simulink model "Senorless"  (R2023a)
settings: Solver=FixedStepDiscrete  StartTime=0.0  StopTime=5  FixedStep=1/FOC_FRQ  RelTol=1e-3
values from neighbouring files (symbols this model uses):
  ADC_REF = 3.6    [Senorless.sldd]
  ADC_SAMPLE_MAX = 32767.0    [Senorless.sldd]
  AMP_GAIN = 16.0    [Senorless.sldd]
  CURR_INPUT = 3276.0    [Senorless.sldd]
  CURR_KI = 380.0    [Senorless.sldd]
  CURR_KP = 0.04    [Senorless.sldd]
  CURR_LIMIT = 0.95    [Senorless.sldd]
  CURR_OVER = 6.0    [Senorless.sldd]
  CURR_POINT_GAIN = 7.0    [Senorless.sldd]
  CURR_STEP = 32760.0    [Senorless.sldd]
  CURR_UNDER = 0.03    [Senorless.sldd]
  CURR_WIDTH = 6552.0    [Senorless.sldd]
  FOC_FRQ = 25000.0    [Senorless.sldd]
  GAMMA = 32767.0    [Senorless.sldd]
  IMAX = 10.0    [Senorless.sldd]
  LPF_FRQ = 2000.0    [Senorless.sldd]
  MOTOR_DAMPER = 2.06E-7    [Senorless.sldd]
  MOTOR_FLUX = 0.00212352    [Senorless.sldd]
  MOTOR_INERTIA = 4.0E-7    [Senorless.sldd]
  MOTOR_LS = 0.000536    [Senorless.sldd]
  MOTOR_PN = 7.0    [Senorless.sldd]
  MOTOR_RS = 4.0    [Senorless.sldd]
  OPEN_IQ = 0.28    [Senorless.sldd]
  OPEN_IQ_MIN = 0.05    [Senorless.sldd]
  OPEN_IQ_SLOW = 0.1    [Senorless.sldd]
  OPEN_SPD = 1000.0    [Senorless.sldd]
  OPEN_SPD_SLOW = 180.0    [Senorless.sldd]
  OPEN_TIME = 0.5    [Senorless.sldd]
  OPEN_TIME_NFO = 0.5    [Senorless.sldd]
  PLL_LIMIT = 0.9    [Senorless.sldd]
  PLL_WIDTH = 800.0    [Senorless.sldd]
  PWM_FRQ = 96000000.0    [Senorless.sldd]
  RS_HUNT = 0.02    [Senorless.sldd]
  SMOK_FRQ = 600.0    [Senorless.sldd]
  SPD_LIMIT = 0.9    [Senorless.sldd]
  SPD_LPF_LEVEL = 0.0    [Senorless.sldd]
  SPD_MAX = 12000.0    [Senorless.sldd]
  SPD_MIN = 4000.0    [Senorless.sldd]
  SPD_REDUCE = 380.0    [Senorless.sldd]
  SPD_STEP = 6.0    [Senorless.sldd]
  SPD_WIDTH = 20.0    [Senorless.sldd]
  THETA_ERR_LIMIT = 8192.0    [Senorless.sldd]
  TS_POINT_GAIN = 10.0    [Senorless.sldd]
  UDC = 48.0    [Senorless.sldd]
  UDC_GAIN = 21.0    [Senorless.sldd]
  UDC_POINT_GAIN = 10.0    [Senorless.sldd]
undefined symbols (not defined in the file or in its folder): curr_q_ki, curr_q_kp, DiscIntNeverNeededParam, magnitude, PLL_LPF_LEVEL, Udc
libraries: simulink x20, slpidlib x5, mcbcontrolslib x2, mcbplantlib x1, autolibpmsmexterior x1, spspowerguiLib x1
(part 6 of 8)

== system Senorless/FOC_PointModel/恒速降力矩强拖/FreqGenerator_point2 ==
  Freq : Inport
  Xo : Inport  Port=2
  Reset : Inport  Port=3
  Data Type Conversion : DataTypeConversion  OutDataTypeStr=int16  SaturateOnIntegerOverflow=off
  Data Type Conversion1 : DataTypeConversion  OutDataTypeStr=int32  SaturateOnIntegerOverflow=off
  Data Type Conversion2 : DataTypeConversion  OutDataTypeStr=int32  SaturateOnIntegerOverflow=off
  Discrete-Time Integrator : DiscreteIntegrator  ExternalReset=falling  InitialConditionSource=external  SampleTime=-1  OutDataTypeStr=int32  RndMeth=Zero  ICPrevOutput=DiscIntNeverNeededParam  ICPrevScaledInput=DiscIntNeverNeededParam
  Gain6 : Gain  Gain=65535  OutDataTypeStr=int32
  MATLAB Function1 : MATLAB Function  Commented=on  TreatAsAtomicUnit=on
  Scope : Scope
  Shift Arithmetic : ArithShift  BitShiftNumber=-8
  Shift Arithmetic1 : ArithShift  BitShiftNumber=8
  Shift Arithmetic2 : ArithShift  BitShiftNumber=-8
  Theta : Outport
  wires:
  Shift Arithmetic/1 -> Discrete-Time Integrator/1
  Freq/1 -> Data Type Conversion1/1
  Gain6/1 -> Shift Arithmetic/1
  Data Type Conversion1/1 -> Gain6/1
  Shift Arithmetic1/1 -> Data Type Conversion/1
  Data Type Conversion/1 -> Theta/1
  Data Type Conversion2/1 -> Shift Arithmetic2/1
  Discrete-Time Integrator/1 -> Scope/1, Shift Arithmetic1/1
  Xo/1 -> Data Type Conversion2/1
  Shift Arithmetic2/1 -> Discrete-Time Integrator/3
  Reset/1 -> Discrete-Time Integrator/2

== system Senorless/FOC_PointModel/恒速降力矩强拖/积分器 ==
  input : Inport
  Xo : Inport  Port=2
  Constant : Constant  OutDataTypeStr=int16
  Data Store Read1 : DataStoreRead  DataStoreName=Ts_Point  IndexOptions=Index vector (dialog)  Indices=1  OutputSizes=1
  Delay : Delay  DelayLength=1  InitialConditionSource=Input port
      settings: InputPortMap=u0,p4
  Product1 : Product  OutDataTypeStr=int32  RndMeth=Zero
  Product2 : Product  OutDataTypeStr=int32  RndMeth=Zero
  Shift Arithmetic : ArithShift  BitShiftNumberSource=Input port  BitShiftNumber=8  BitShiftDirection=Right
      settings: InputPortMap=u0,p1
  Sum : Sum  Inputs=|++  OutDataTypeStr=int32  RndMeth=Zero
  周期定点化适当放大2^n : Constant  Value=TS_POINT_GAIN
  这个是缩小周期增益的 : ArithShift  BitShiftNumber=15  DiagnosticForOORShift=Error
  output : Outport
  wires:
  Sum/1 -> Delay/1, output/1
  Product2/1 -> 这个是缩小周期增益的/1
  input/1 -> Shift Arithmetic/1
  Data Store Read1/1 -> Product2/1
  Shift Arithmetic/1 -> Product2/2
  周期定点化适当放大2^n/1 -> Shift Arithmetic/2
  Xo/1 -> Delay/2
  这个是缩小周期增益的/1 -> Product1/1
  Constant/1 -> Product1/2
  Product1/1 -> Sum/1
  Delay/1 -> Sum/2

== system Senorless/FOC_PointModel/慢速开环/FreqGenerator_point2 ==
  Freq : Inport
  Xo : Inport  Port=2
  Reset : Inport  Port=3
  Data Type Conversion : DataTypeConversion  OutDataTypeStr=int16  SaturateOnIntegerOverflow=off
  Data Type Conversion1 : DataTypeConversion  OutDataTypeStr=int32  SaturateOnIntegerOverflow=off
  Data Type Conversion2 : DataTypeConversion  OutDataTypeStr=int32  SaturateOnIntegerOverflow=off
  Discrete-Time Integrator : DiscreteIntegrator  ExternalReset=falling  InitialConditionSource=external  SampleTime=-1  OutDataTypeStr=int32  RndMeth=Zero  ICPrevOutput=DiscIntNeverNeededParam  ICPrevScaledInput=DiscIntNeverNeededParam
  Gain6 : Gain  Gain=65535  OutDataTypeStr=int32
  MATLAB Function1 : MATLAB Function  Commented=on  TreatAsAtomicUnit=on
  Scope : Scope
  Shift Arithmetic : ArithShift  BitShiftNumber=-8
  Shift Arithmetic1 : ArithShift  BitShiftNumber=8
  Shift Arithmetic2 : ArithShift  BitShiftNumber=-8
  Theta : Outport
  wires:
  Reset/1 -> Discrete-Time Integrator/2
  Shift Arithmetic2/1 -> Discrete-Time Integrator/3
  Xo/1 -> Data Type Conversion2/1
  Discrete-Time Integrator/1 -> Shift Arithmetic1/1, Scope/1
  Data Type Conversion2/1 -> Shift Arithmetic2/1
  Data Type Conversion/1 -> Theta/1
  Shift Arithmetic1/1 -> Data Type Conversion/1
  Data Type Conversion1/1 -> Gain6/1
  Gain6/1 -> Shift Arithmetic/1
  Freq/1 -> Data Type Conversion1/1
  Shift Arithmetic/1 -> Discrete-Time Integrator/1

== system Senorless/FOC_PointModel/慢速开环/积分器 ==
  input : Inport
  Constant : Constant  OutDataTypeStr=int16
  Data Store Read1 : DataStoreRead  DataStoreName=Ts_Point  IndexOptions=Index vector (dialog)  Indices=1  OutputSizes=1
  Product1 : Product  OutDataTypeStr=int32  RndMeth=Zero
  Product2 : Product  OutDataTypeStr=int32  RndMeth=Zero
  Shift Arithmetic : ArithShift  BitShiftNumberSource=Input port  BitShiftNumber=8  BitShiftDirection=Right
      settings: InputPortMap=u0,p1
  Sum : Sum  Inputs=|++  OutDataTypeStr=int32  RndMeth=Zero
  Unit Delay : UnitDelay  SampleTime=-1  HasFrameUpgradeWarning=on
  周期定点化适当放大2^n : Constant  Value=TS_POINT_GAIN
  这个是缩小周期增益的 : ArithShift  BitShiftNumber=15  DiagnosticForOORShift=Error
  output : Outport
  wires:
  周期定点化适当放大2^n/1 -> Shift Arithmetic/2
  Shift Arithmetic/1 -> Product2/2
  Data Store Read1/1 -> Product2/1
  input/1 -> Shift Arithmetic/1
  这个是缩小周期增益的/1 -> Product1/2
  Product2/1 -> 这个是缩小周期增益的/1
  Product1/1 -> Sum/1
  Sum/1 -> Unit Delay/1, output/1
  Unit Delay/1 -> Sum/2
  Constant/1 -> Product1/1

== system Senorless/FOC_PointModel/观测器闭环//速度环/PI Controller ==
  input : Inport
  Kp : Inport  Port=2
  Ki : Inport  Port=3
  Data Store Read3 : DataStoreRead  DataStoreName=Speed_Limit  IndexOptions=Index vector (dialog)  Indices=1  OutputSizes=1
  Gain : Gain  Gain=-1  OutDataTypeStr=int32  RndMeth=Zero
  Product2 : Product  OutDataTypeStr=int32  RndMeth=Zero
  Saturation Dynamic2 : simulink/Discontinuities/Saturation Dynamic  OutMin=[]  OutMax=[]  OutDataTypeStr=Inherit: Same as second input  OutDataType=fixdt(1, 16)  OutScaling=2^-10  RndMeth=Zero  DoSatur=off
  Scope : Scope  NumInputPorts=2
  Scope1 : Scope  NumInputPorts=2
  Sum : Sum  OutDataTypeStr=int32  RndMeth=Zero
  input1 : InportShadow
  积分器 : Subsystem  Commented=on
      settings: MinAlgLoopOccurrences=on
  output : Outport
  wires:
  input/1 -> Scope1/1, Product2/1
  input1/1 -> 积分器/2(input)
  Sum/1 -> Saturation Dynamic2/2
  Saturation Dynamic2/1 -> output/1
  Data Store Read3/1 -> [limit]
  [limit] -> Gain/1
  Product2/1 -> Scope1/2, Sum/1, Scope/1
  积分器/1(output) -> Scope/2
  Kp/1 -> Product2/2
  Ki/1 -> 积分器/1(Ki)
  Gain/1 -> Saturation Dynamic2/3
  [limit] -> Saturation Dynamic2/1

== system Senorless/FOC_PointModel/观测器闭环//速度环/积分器//上升沿初始化 ==
  Ki : Inport
  input : Inport  Port=2
  Reset : Inport  Port=3
  Xo : Inport  Port=4
  Data Store Memory : DataStoreMemory  DataStoreName=tmp  WriteAfterWriteMsg=warning  ShowAdditionalParam=off  OutDataTypeStr=int32
  Data Store Read : DataStoreRead  DataStoreName=tmp  IndexOptions=Index vector (dialog)  Indices=1  OutputSizes=1
  Data Store Read1 : DataStoreRead  DataStoreName=Ts_Point  IndexOptions=Index vector (dialog)  Indices=1  OutputSizes=1
  Data Store Write : DataStoreWrite  DataStoreName=tmp  IndexOptions=Index vector (dialog)  Indices=1  OutputSizes=1
  Data Type Conversion2 : DataTypeConversion  OutDataTypeStr=int32  SaturateOnIntegerOverflow=off
  Data Type Conversion3 : DataTypeConversion  Commented=on  OutDataTypeStr=int16  SaturateOnIntegerOverflow=off
  Divide : Product  Commented=on  Inputs=*/  OutDataTypeStr=int32  RndMeth=Zero
  MATLAB Function : MATLAB Function  TreatAsAtomicUnit=on
  Product1 : Product  OutDataTypeStr=int32  RndMeth=Zero
  Product2 : Product  OutDataTypeStr=int32  RndMeth=Zero
  Reset_Block : Subsystem
  Scope : Scope
  Sum : Sum  Inputs=|++  OutDataTypeStr=int32  RndMeth=Zero
  Sum1 : Sum  Inputs=|+-  OutDataTypeStr=int32  RndMeth=Zero
  Ts适当放大的缩小系数， 详见初始化模块 : ArithShift  Commented=on  BitShiftNumber=TS_POINT_GAIN  DiagnosticForOORShift=Error
  Unit Delay : UnitDelay  SampleTime=-1  HasFrameUpgradeWarning=on
  周期定点化适当放大2^n : Constant  Value=TS_POINT_GAIN
  积分器运行频率 : Constant  Commented=on  Value=FOC_FRQ
  这个是缩小周期增益的 : ArithShift  BitShiftNumber=15  DiagnosticForOORShift=Error
  output : Outport
  wires:
  周期定点化适当放大2^n/1 -> MATLAB Function/2(n)
  Sum1/1 -> Reset_Block/1(Xo)
  MATLAB Function/1(out) -> Product2/2
  Data Store Read1/1 -> Product2/1
  input/1 -> MATLAB Function/1(in)
  这个是缩小周期增益的/1 -> Product1/2
  Product2/1 -> 这个是缩小周期增益的/1
  Data Type Conversion3/1 -> Divide/2
  Ki/1 -> Product1/1
  Xo/1 -> Data Type Conversion2/1
  积分器运行频率/1 -> Data Type Conversion3/1
  Product1/1 -> Sum/1, Sum1/2
  Data Type Conversion2/1 -> Sum1/1
  Unit Delay/1 -> Data Store Write/1
  Sum/1 -> output/1, Scope/1, Unit Delay/1
  Data Store Read/1 -> Sum/2
  Reset/1 -> Reset_Block/Trigger

== system Senorless/FOC_PointModel/Err/闭环错误判断/SUM ==
  in : Inport
  Action Port : ActionPort  InitializeStates=reset  ActionPortLabel=if(u1 > 0)
  Sum : Sum  Inputs=|++  OutDataTypeStr=int32  RndMeth=Zero
  Unit Delay2 : UnitDelay  SampleTime=-1  HasFrameUpgradeWarning=on
  out : Outport
  wires:
  Sum/1 -> Unit Delay2/1
  in/1 -> Sum/1
  Unit Delay2/1 -> out/1, Sum/2

== system Senorless/FOC_PointModel/Err/闭环错误判断/ZERO ==
  Action Port : ActionPort  InitializeStates=reset  ActionPortLabel=else
  Constant : Constant  Value=0  OutDataTypeStr=int32
  out : Outport
  wires:
  Constant/1 -> out/1

== system Senorless/FOC_PointModel/Observers/PLL/LPF ==
  note: a =(ω c​ T s​ )/(1+ω c​ T s​ )
  note: y(n)=ax(n)+(1−a)y(n−1)
  input : Inport
  Constant1 : Constant  Value=SPD_LPF_LEVEL  OutDataTypeStr=int16
  Constant5 : Constant  OutDataTypeStr=int16
  Product10 : Product  OutDataTypeStr=int32
  Product11 : Product  OutDataTypeStr=int32  RndMeth=Zero
  Saturation : Saturate  UpperLimit=15  LowerLimit=0  RndMeth=Zero
  Shift Arithmetic1 : ArithShift  BitShiftNumber=-4
  Shift Arithmetic9 : ArithShift  BitShiftNumber=4
  Sum10 : Sum  Inputs=-+
  Sum11 : Sum  OutDataTypeStr=int32  RndMeth=Zero
  Unit Delay9 : UnitDelay  SampleTime=-1  HasFrameUpgradeWarning=on
  output : Outport
  wires:
  Constant1/1 -> Saturation/1
  Constant5/1 -> Shift Arithmetic1/1
  Sum11/1 -> Shift Arithmetic9/1
  Shift Arithmetic9/1 -> output/1, Unit Delay9/1
  Shift Arithmetic1/1 -> Sum10/2
  Sum10/1 -> Product10/1
  Product11/1 -> Sum11/1
  Product10/1 -> Sum11/2
  Unit Delay9/1 -> Product11/1
  input/1 -> Product10/2
  Saturation/1 -> Sum10/1, Product11/2

== system Senorless/FOC_PointModel/Observers/PLL/PI Controller ==
  input : Inport
  Kp : Inport  Port=2
  Ki : Inport  Port=3
  Data Store Read3 : DataStoreRead  DataStoreName=PLL_Limit  IndexOptions=Index vector (dialog)  Indices=1  OutputSizes=1
  Gain : Gain  Gain=-1  OutDataTypeStr=int32  RndMeth=Zero
  Product2 : Product  OutDataTypeStr=int32  RndMeth=Zero
  Saturation Dynamic2 : simulink/Discontinuities/Saturation Dynamic  OutMin=[]  OutMax=[]  OutDataTypeStr=Inherit: Same as second input  OutDataType=fixdt(1, 16)  OutScaling=2^-10  RndMeth=Zero  DoSatur=off
  Scope : Scope  NumInputPorts=2
  Sum : Sum  OutDataTypeStr=int32  RndMeth=Zero
  input1 : InportShadow
  积分器 : Subsystem
      settings: MinAlgLoopOccurrences=on
  output : Outport
  wires:
  input/1 -> Product2/1
  Kp/1 -> Product2/2
  Ki/1 -> 积分器/1(Ki)
  input1/1 -> 积分器/2(input)
  Product2/1 -> Sum/1, Scope/1
  积分器/1(output) -> Scope/2, Sum/2
  Saturation Dynamic2/1 -> output/1
  Data Store Read3/1 -> [Limit]
  [Limit] -> Gain/1
  Gain/1 -> Saturation Dynamic2/3
  Sum/1 -> Saturation Dynamic2/2
  [Limit] -> Saturation Dynamic2/1

== system Senorless/FOC_PointModel/Observers/PLL/PLL_LPF1 ==
  note: y(n)=ax(n)+(1−a)y(n−1)
  note: a =(ω c​ T s​ )/(1+ω c​ T s​ )
  input : Inport
  Constant1 : Constant  Value=PLL_LPF_LEVEL  OutDataTypeStr=int16
  Constant5 : Constant  OutDataTypeStr=int16
  Product10 : Product  OutDataTypeStr=int32
  Product11 : Product  OutDataTypeStr=int32  RndMeth=Zero
  Shift Arithmetic1 : ArithShift  BitShiftNumber=-4
  Shift Arithmetic9 : ArithShift  BitShiftNumber=4
  Sum10 : Sum  Inputs=-+
  Sum11 : Sum  OutDataTypeStr=int32  RndMeth=Zero
  Unit Delay9 : UnitDelay  SampleTime=-1  HasFrameUpgradeWarning=on
  output : Outport
  wires:
  input/1 -> Product10/2
  Unit Delay9/1 -> Product11/1
  Product10/1 -> Sum11/2
  Product11/1 -> Sum11/1
  Sum10/1 -> Product10/1
  Shift Arithmetic1/1 -> Sum10/2
  Shift Arithmetic9/1 -> Unit Delay9/1, output/1
  Sum11/1 -> Shift Arithmetic9/1
  Constant5/1 -> Shift Arithmetic1/1
  Constant1/1 -> Product11/2, Sum10/1

== system Senorless/FOC_PointModel/Observers/PLL/sincos_512 ==
  theta : Inport
  Constant3 : Constant  Value=16384  OutDataTypeStr=uint16
  Shift Arithmetic : ArithShift  BitShiftNumber=7
  Shift Arithmetic1 : ArithShift  BitShiftNumber=7
  Sin : Lookup_n-D  NumberOfTableDimensions=1  BreakpointsSpecification=Even spacing  BreakpointsForDimension1=uint16(linspace(0,511,512))  BreakpointsForDimension1DataTypeStr=uint16  IndexSearchMethod=Linear search  BeginIndexSearchUsingPreviousIndexResult=on  UseOneInputPortForAllInputData=on  Table=int16(32767*sin(linspace(0,2*pi,512)))  TableDataTypeStr=int16  IntermediateResultsDataTypeStr=int32  InterpMethod=Flat  ExtrapMethod=Clip  RemoveProtectionInput=on  ApplyFullPrecisionForLinearInterpolation=on  InternalRulePriority=Speed  OutDataTypeStr=int16  RndMeth=Zero  FractionDataTypeStr=fixdt(1,16,0)  InputSameDT=off
  Sin1 : Lookup_n-D  NumberOfTableDimensions=1  BreakpointsSpecification=Even spacing  BreakpointsForDimension1=uint16(linspace(0,511,512))  BreakpointsForDimension1DataTypeStr=uint16  IndexSearchMethod=Linear search  BeginIndexSearchUsingPreviousIndexResult=on  UseOneInputPortForAllInputData=on  Table=int16(32767*sin(linspace(0,2*pi,512)))  TableDataTypeStr=int16  IntermediateResultsDataTypeStr=int32  InterpMethod=Flat  ExtrapMethod=Clip  RemoveProtectionInput=on  ApplyFullPrecisionForLinearInterpolation=on  InternalRulePriority=Speed  OutDataTypeStr=int16  RndMeth=Zero  FractionDataTypeStr=fixdt(1,16,0)  InputSameDT=off
  Sum2 : Sum  Inputs=|++
  theta1 : InportShadow
  cos : Outport
  sin : Outport  Port=2
  wires:
  Sin1/1 -> cos/1
  Sin/1 -> sin/1
  Shift Arithmetic/1 -> Sin1/1
  Sum2/1 -> Shift Arithmetic/1
  Constant3/1 -> Sum2/2
  Shift Arithmetic1/1 -> Sin/1
  theta1/1 -> Sum2/1
  theta/1 -> Shift Arithmetic1/1

== system Senorless/FOC_PointModel/Observers/PLL/积分器 ==
  input : Inport
  Constant : Constant  OutDataTypeStr=int16
  Data Store Read1 : DataStoreRead  DataStoreName=Ts_Point  IndexOptions=Index vector (dialog)  Indices=1  OutputSizes=1
  Data Type Conversion3 : DataTypeConversion  Commented=on  OutDataTypeStr=int16  SaturateOnIntegerOverflow=off
  Divide : Product  Commented=on  Inputs=*/  OutDataTypeStr=int32  RndMeth=Zero
  Product1 : Product  OutDataTypeStr=int32  RndMeth=Zero
  Product2 : Product  OutDataTypeStr=int32  RndMeth=Zero
  Shift Arithmetic : ArithShift  BitShiftNumberSource=Input port  BitShiftNumber=8  BitShiftDirection=Right
      settings: InputPortMap=u0,p1
  Sum : Sum  Inputs=|++  OutDataTypeStr=int32  RndMeth=Zero
  Ts适当放大的缩小系数， 详见初始化模块 : ArithShift  Commented=on  BitShiftNumber=TS_POINT_GAIN  DiagnosticForOORShift=Error
  Unit Delay : UnitDelay  SampleTime=-1  HasFrameUpgradeWarning=on
  周期定点化适当放大2^n : Constant  Value=TS_POINT_GAIN
  积分器运行频率 : Constant  Commented=on  Value=FOC_FRQ
  这个是缩小周期增益的 : ArithShift  BitShiftNumber=15  DiagnosticForOORShift=Error
  output : Outport
  wires:
  积分器运行频率/1 -> Data Type Conversion3/1
  Data Type Conversion3/1 -> Divide/2
  周期定点化适当放大2^n/1 -> Shift Arithmetic/2
  Sum/1 -> output/1, Unit Delay/1
  Unit Delay/1 -> Sum/2
  input/1 -> Shift Arithmetic/1
  Shift Arithmetic/1 -> Product2/2
  Data Store Read1/1 -> Product2/1
  Product2/1 -> 这个是缩小周期增益的/1
  这个是缩小周期增益的/1 -> Product1/2
  Constant/1 -> Product1/1
  Product1/1 -> Sum/1

== system Senorless/FOC_PointModel/Observers/PLL2/LPF ==
  note: y(n)=ax(n)+(1−a)y(n−1)
  note: a =(ω c​ T s​ )/(1+ω c​ T s​ )
  input : Inport
  Constant1 : Constant  Value=8  OutDataTypeStr=int16
  Constant5 : Constant  OutDataTypeStr=int16
  Product10 : Product  OutDataTypeStr=int32
  Product11 : Product  OutDataTypeStr=int32  RndMeth=Zero
  Saturation : Saturate  UpperLimit=15  LowerLimit=0  RndMeth=Zero
  Shift Arithmetic1 : ArithShift  BitShiftNumber=-4
  Shift Arithmetic9 : ArithShift  BitShiftNumber=4
  Sum10 : Sum  Inputs=-+
  Sum11 : Sum  OutDataTypeStr=int32  RndMeth=Zero
  Unit Delay9 : UnitDelay  SampleTime=-1  HasFrameUpgradeWarning=on
  output : Outport
  wires:
  Saturation/1 -> Product11/2, Sum10/1
  input/1 -> Product10/2
  Unit Delay9/1 -> Product11/1
  Product10/1 -> Sum11/2
  Product11/1 -> Sum11/1
  Sum10/1 -> Product10/1
  Shift Arithmetic1/1 -> Sum10/2
  Shift Arithmetic9/1 -> Unit Delay9/1, output/1
  Sum11/1 -> Shift Arithmetic9/1
  Constant5/1 -> Shift Arithmetic1/1
  Constant1/1 -> Saturation/1

== system Senorless/FOC_PointModel/Observers/PLL2/PI Controller ==
  input : Inport
  Kp : Inport  Port=2
  Ki : Inport  Port=3
  Data Store Read3 : DataStoreRead  DataStoreName=PLL_Limit  IndexOptions=Index vector (dialog)  Indices=1  OutputSizes=1
  Gain : Gain  Gain=-1  OutDataTypeStr=int32  RndMeth=Zero
  Product2 : Product  OutDataTypeStr=int32  RndMeth=Zero
  Saturation Dynamic2 : simulink/Discontinuities/Saturation Dynamic  OutMin=[]  OutMax=[]  OutDataTypeStr=Inherit: Same as second input  OutDataType=fixdt(1, 16)  OutScaling=2^-10  RndMeth=Zero  DoSatur=off
  Scope : Scope  NumInputPorts=2
  Sum : Sum  OutDataTypeStr=int32  RndMeth=Zero
  input1 : InportShadow
  积分器 : Subsystem
      settings: MinAlgLoopOccurrences=on
  output : Outport
  wires:
  [Limit] -> Saturation Dynamic2/1
  Sum/1 -> Saturation Dynamic2/2
  Gain/1 -> Saturation Dynamic2/3
  [Limit] -> Gain/1
  Data Store Read3/1 -> [Limit]
  Saturation Dynamic2/1 -> output/1
  积分器/1(output) -> Sum/2, Scope/2
  Product2/1 -> Scope/1, Sum/1
  input1/1 -> 积分器/2(input)
  Ki/1 -> 积分器/1(Ki)
  Kp/1 -> Product2/2
  input/1 -> Product2/1

== system Senorless/FOC_PointModel/Observers/PLL2/PLL_LPF1 ==
  note: a =(ω c​ T s​ )/(1+ω c​ T s​ )
  note: y(n)=ax(n)+(1−a)y(n−1)
  input : Inport
  Constant1 : Constant  Value=PLL_LPF_LEVEL  OutDataTypeStr=int16
  Constant5 : Constant  OutDataTypeStr=int16
  Product10 : Product  OutDataTypeStr=int32
  Product11 : Product  OutDataTypeStr=int32  RndMeth=Zero
  Shift Arithmetic1 : ArithShift  BitShiftNumber=-4
  Shift Arithmetic9 : ArithShift  BitShiftNumber=4
  Sum10 : Sum  Inputs=-+
  Sum11 : Sum  OutDataTypeStr=int32  RndMeth=Zero
  Unit Delay9 : UnitDelay  SampleTime=-1  HasFrameUpgradeWarning=on
  output : Outport
  wires:
  Constant1/1 -> Sum10/1, Product11/2
  Constant5/1 -> Shift Arithmetic1/1
  Sum11/1 -> Shift Arithmetic9/1
  Shift Arithmetic9/1 -> output/1, Unit Delay9/1
  Shift Arithmetic1/1 -> Sum10/2
  Sum10/1 -> Product10/1
  Product11/1 -> Sum11/1
  Product10/1 -> Sum11/2
  Unit Delay9/1 -> Product11/1
  input/1 -> Product10/2

== system Senorless/FOC_PointModel/Observers/PLL2/sincos_512 ==
  theta : Inport
  Constant3 : Constant  Value=16384  OutDataTypeStr=uint16
  Shift Arithmetic : ArithShift  BitShiftNumber=7
  Shift Arithmetic1 : ArithShift  BitShiftNumber=7
  Sin : Lookup_n-D  NumberOfTableDimensions=1  BreakpointsSpecification=Even spacing  BreakpointsForDimension1=uint16(linspace(0,511,512))  BreakpointsForDimension1DataTypeStr=uint16  IndexSearchMethod=Linear search  BeginIndexSearchUsingPreviousIndexResult=on  UseOneInputPortForAllInputData=on  Table=int16(32767*sin(linspace(0,2*pi,512)))  TableDataTypeStr=int16  IntermediateResultsDataTypeStr=int32  InterpMethod=Flat  ExtrapMethod=Clip  RemoveProtectionInput=on  ApplyFullPrecisionForLinearInterpolation=on  InternalRulePriority=Speed  OutDataTypeStr=int16  RndMeth=Zero  FractionDataTypeStr=fixdt(1,16,0)  InputSameDT=off
  Sin1 : Lookup_n-D  NumberOfTableDimensions=1  BreakpointsSpecification=Even spacing  BreakpointsForDimension1=uint16(linspace(0,511,512))  BreakpointsForDimension1DataTypeStr=uint16  IndexSearchMethod=Linear search  BeginIndexSearchUsingPreviousIndexResult=on  UseOneInputPortForAllInputData=on  Table=int16(32767*sin(linspace(0,2*pi,512)))  TableDataTypeStr=int16  IntermediateResultsDataTypeStr=int32  InterpMethod=Flat  ExtrapMethod=Clip  RemoveProtectionInput=on  ApplyFullPrecisionForLinearInterpolation=on  InternalRulePriority=Speed  OutDataTypeStr=int16  RndMeth=Zero  FractionDataTypeStr=fixdt(1,16,0)  InputSameDT=off
  Sum2 : Sum  Inputs=|++
  theta1 : InportShadow
  cos : Outport
  sin : Outport  Port=2
  wires:
  theta/1 -> Shift Arithmetic1/1
  theta1/1 -> Sum2/1
  Shift Arithmetic1/1 -> Sin/1
  Constant3/1 -> Sum2/2
  Sum2/1 -> Shift Arithmetic/1
  Shift Arithmetic/1 -> Sin1/1
  Sin/1 -> sin/1
  Sin1/1 -> cos/1

== system Senorless/FOC_PointModel/Observers/PLL2/积分器 ==
  input : Inport
  Constant : Constant  OutDataTypeStr=int16
  Data Store Read1 : DataStoreRead  DataStoreName=Ts_Point  IndexOptions=Index vector (dialog)  Indices=1  OutputSizes=1
  Data Type Conversion3 : DataTypeConversion  Commented=on  OutDataTypeStr=int16  SaturateOnIntegerOverflow=off
  Divide : Product  Commented=on  Inputs=*/  OutDataTypeStr=int32  RndMeth=Zero
  Product1 : Product  OutDataTypeStr=int32  RndMeth=Zero
  Product2 : Product  OutDataTypeStr=int32  RndMeth=Zero
  Shift Arithmetic : ArithShift  BitShiftNumberSource=Input port  BitShiftNumber=8  BitShiftDirection=Right
      settings: InputPortMap=u0,p1
  Sum : Sum  Inputs=|++  OutDataTypeStr=int32  RndMeth=Zero
  Ts适当放大的缩小系数， 详见初始化模块 : ArithShift  Commented=on  BitShiftNumber=TS_POINT_GAIN  DiagnosticForOORShift=Error
  Unit Delay : UnitDelay  SampleTime=-1  HasFrameUpgradeWarning=on
  周期定点化适当放大2^n : Constant  Value=TS_POINT_GAIN
  积分器运行频率 : Constant  Commented=on  Value=FOC_FRQ
  这个是缩小周期增益的 : ArithShift  BitShiftNumber=15  DiagnosticForOORShift=Error
  output : Outport
  wires:
  Product1/1 -> Sum/1
  Constant/1 -> Product1/1
  这个是缩小周期增益的/1 -> Product1/2
  Product2/1 -> 这个是缩小周期增益的/1
  Data Store Read1/1 -> Product2/1
  Shift Arithmetic/1 -> Product2/2
  input/1 -> Shift Arithmetic/1
  Unit Delay/1 -> Sum/2
  Sum/1 -> Unit Delay/1, output/1
  周期定点化适当放大2^n/1 -> Shift Arithmetic/2
  Data Type Conversion3/1 -> Divide/2
  积分器运行频率/1 -> Data Type Conversion3/1

== system Senorless/FOC_PointModel/Observers/SMO/SMO_LPF1 ==
  note: y(n)=ax(n)+(1−a)y(n−1)
  note: a =(ω c​ T s​ )/(1+ω c​ T s​ )
  input : Inport
  Constant5 : Constant  Value=32767  OutDataTypeStr=int16
  Data Store Read1 : DataStoreRead  DataStoreName=LPF_FRQ_Point  IndexOptions=Index vector (dialog)  Indices=1  OutputSizes=1
  Data Store Read7 : DataStoreRead  DataStoreName=LPF_FRQ_Point  IndexOptions=Index vector (dialog)  Indices=1  OutputSizes=1
  Product1 : Product  OutDataTypeStr=int32  RndMeth=Zero
  Product10 : Product  OutDataTypeStr=int32
  Product11 : Product  OutDataTypeStr=int32  RndMeth=Zero
  Shift Arithmetic2 : ArithShift  BitShiftNumber=15
  Shift Arithmetic3 : ArithShift  BitShiftNumber=15
  Shift Arithmetic4 : ArithShift  BitShiftNumber=15
  Sum1 : Sum  Inputs=-+  OutDataTypeStr=int32  RndMeth=Zero
  Sum10 : Sum  Inputs=-+  OutDataTypeStr=int16  RndMeth=Zero
  Sum11 : Sum  OutDataTypeStr=int32  RndMeth=Zero
  Sum2 : Sum  OutDataTypeStr=int32  RndMeth=Zero
  Unit Delay1 : UnitDelay  SampleTime=-1  HasFrameUpgradeWarning=on
  Unit Delay9 : UnitDelay  SampleTime=-1  HasFrameUpgradeWarning=on
  input1 : InportShadow
  output : Outport
  wires:
  Product10/1 -> Shift Arithmetic3/1
  Product11/1 -> Shift Arithmetic2/1
  Unit Delay9/1 -> Product10/2
  Sum10/1 -> Product10/1
  input/1 -> Product11/1
  Data Store Read7/1 -> Sum10/1, Product11/2
  Sum11/1 -> Unit Delay9/1
  Shift Arithmetic2/1 -> Sum11/1
  Shift Arithmetic3/1 -> Sum11/2
  input1/1 -> Sum1/2
  Unit Delay1/1 -> Sum2/1, Sum1/1
  Sum2/1 -> output/1, Unit Delay1/1
  Sum1/1 -> Product1/1
  Data Store Read1/1 -> Product1/2
  Product1/1 -> Shift Arithmetic4/1
  Shift Arithmetic4/1 -> Sum2/2
  Constant5/1 -> Sum10/2

== system Senorless/FOC_PointModel/Observers/SMO/SMO_LPF2 ==
  note: a =(ω c​ T s​ )/(1+ω c​ T s​ )
  note: y(n)=ax(n)+(1−a)y(n−1)
  input : Inport
  Constant5 : Constant  Value=32767  OutDataTypeStr=int16
  Data Store Read1 : DataStoreRead  DataStoreName=LPF_FRQ_Point  IndexOptions=Index vector (dialog)  Indices=1  OutputSizes=1
  Data Store Read7 : DataStoreRead  DataStoreName=LPF_FRQ_Point  IndexOptions=Index vector (dialog)  Indices=1  OutputSizes=1
  Product1 : Product  OutDataTypeStr=int32  RndMeth=Zero
  Product10 : Product  OutDataTypeStr=int32
  Product11 : Product  OutDataTypeStr=int32  RndMeth=Zero
  Shift Arithmetic2 : ArithShift  BitShiftNumber=15
  Shift Arithmetic3 : ArithShift  BitShiftNumber=15
  Shift Arithmetic4 : ArithShift  BitShiftNumber=15
  Sum1 : Sum  Inputs=-+  OutDataTypeStr=int32  RndMeth=Zero
  Sum10 : Sum  Inputs=-+  OutDataTypeStr=int16  RndMeth=Zero
  Sum11 : Sum  OutDataTypeStr=int32  RndMeth=Zero
  Sum2 : Sum  OutDataTypeStr=int32  RndMeth=Zero
  Unit Delay1 : UnitDelay  SampleTime=-1  HasFrameUpgradeWarning=on
  Unit Delay9 : UnitDelay  SampleTime=-1  HasFrameUpgradeWarning=on
  input1 : InportShadow
  output : Outport
  wires:
  Shift Arithmetic4/1 -> Sum2/2
  Product1/1 -> Shift Arithmetic4/1
  Data Store Read1/1 -> Product1/2
  Sum1/1 -> Product1/1
  Sum2/1 -> output/1, Unit Delay1/1
  Unit Delay1/1 -> Sum1/1, Sum2/1
  input1/1 -> Sum1/2
  Shift Arithmetic3/1 -> Sum11/2
  Shift Arithmetic2/1 -> Sum11/1
  Data Store Read7/1 -> Product11/2, Sum10/1
  Constant5/1 -> Sum10/2
  input/1 -> Product11/1
  Sum10/1 -> Product10/1
  Unit Delay9/1 -> Product10/2
  Product11/1 -> Shift Arithmetic2/1
  Product10/1 -> Shift Arithmetic3/1
  Sum11/1 -> Unit Delay9/1

== system Senorless/FOC_PointModel/Observers/SMO/SMO_LPF4 ==
  note: a =(ω c​ T s​ )/(1+ω c​ T s​ )
  note: y(n)=ax(n)+(1−a)y(n−1)
  input : Inport
  Constant5 : Constant  OutDataTypeStr=int16
  Data Store Read7 : DataStoreRead  DataStoreName=LPF_FRQ_Point  IndexOptions=Index vector (dialog)  Indices=1  OutputSizes=1
  Data Type Conversion6 : DataTypeConversion  OutDataTypeStr=int16  SaturateOnIntegerOverflow=off
  Product10 : Product  OutDataTypeStr=int32
  Product11 : Product  OutDataTypeStr=int32  RndMeth=Zero
  Shift Arithmetic1 : ArithShift  BitShiftNumber=-4
  Shift Arithmetic9 : ArithShift  BitShiftNumber=4
  Sum10 : Sum  Inputs=-+
  Sum11 : Sum  OutDataTypeStr=int32  RndMeth=Zero
  Unit Delay9 : UnitDelay  SampleTime=-1  HasFrameUpgradeWarning=on
  output : Outport
  wires:
  Constant5/1 -> Shift Arithmetic1/1
  Sum11/1 -> Shift Arithmetic9/1
  Data Type Conversion6/1 -> output/1, Unit Delay9/1
  Shift Arithmetic9/1 -> Data Type Conversion6/1
  Data Store Read7/1 -> Product11/2, Sum10/1
  Shift Arithmetic1/1 -> Sum10/2
  input/1 -> Product11/1
  Sum10/1 -> Product10/1
  Unit Delay9/1 -> Product10/2
  Product11/1 -> Sum11/1
  Product10/1 -> Sum11/2

== system Senorless/FOC_PointModel/Observers/SMO/SMO_LPF5 ==
  note: y(n)=ax(n)+(1−a)y(n−1)
  note: a =(ω c​ T s​ )/(1+ω c​ T s​ )
  input : Inport
  Constant5 : Constant  OutDataTypeStr=int16
  Data Store Read7 : DataStoreRead  DataStoreName=LPF_FRQ_Point  IndexOptions=Index vector (dialog)  Indices=1  OutputSizes=1
  Data Type Conversion6 : DataTypeConversion  OutDataTypeStr=int16  SaturateOnIntegerOverflow=off
  Product10 : Product  OutDataTypeStr=int32
  Product11 : Product  OutDataTypeStr=int32  RndMeth=Zero
  Shift Arithmetic1 : ArithShift  BitShiftNumber=-4
  Shift Arithmetic9 : ArithShift  BitShiftNumber=4
  Sum10 : Sum  Inputs=-+
  Sum11 : Sum  OutDataTypeStr=int32  RndMeth=Zero
  Unit Delay9 : UnitDelay  SampleTime=-1  HasFrameUpgradeWarning=on
  output : Outport
  wires:
  Product10/1 -> Sum11/2
  Product11/1 -> Sum11/1
  Unit Delay9/1 -> Product10/2
  Sum10/1 -> Product10/1
  input/1 -> Product11/1
  Shift Arithmetic1/1 -> Sum10/2
  Data Store Read7/1 -> Sum10/1, Product11/2
  Shift Arithmetic9/1 -> Data Type Conversion6/1
  Data Type Conversion6/1 -> Unit Delay9/1, output/1
  Sum11/1 -> Shift Arithmetic9/1
  Constant5/1 -> Shift Arithmetic1/1

== system Senorless/FOC_PointModel/Observers/纯浮点NFO/LPF ==
  note: a =(ω c​ T s​ )/(1+ω c​ T s​ )
  note: y(n)=ax(n)+(1−a)y(n−1)
  input : Inport
  Constant1 : Constant  Value=SPD_LPF_LEVEL  OutDataTypeStr=int16
  Constant5 : Constant  OutDataTypeStr=int16
  Product10 : Product  OutDataTypeStr=int32
  Product11 : Product  OutDataTypeStr=int32  RndMeth=Zero
  Saturation : Saturate  UpperLimit=15  LowerLimit=0  RndMeth=Zero
  Shift Arithmetic1 : ArithShift  BitShiftNumber=-4
  Shift Arithmetic9 : ArithShift  BitShiftNumber=4
  Sum10 : Sum  Inputs=-+
  Sum11 : Sum  OutDataTypeStr=int32  RndMeth=Zero
  Unit Delay9 : UnitDelay  SampleTime=-1  HasFrameUpgradeWarning=on
  output : Outport
  wires:
  Constant1/1 -> Saturation/1
  Constant5/1 -> Shift Arithmetic1/1
  Sum11/1 -> Shift Arithmetic9/1
  Shift Arithmetic9/1 -> output/1, Unit Delay9/1
  Shift Arithmetic1/1 -> Sum10/2
  Sum10/1 -> Product10/1
  Product11/1 -> Sum11/1
  Product10/1 -> Sum11/2
  Unit Delay9/1 -> Product11/1
  input/1 -> Product10/2
  Saturation/1 -> Sum10/1, Product11/2

== system Senorless/FOC_PointModel/idq_Controller/PI Controller/积分器 ==
  Ki : Inport
  input : Inport  Port=2
  Constant : Constant  Value=32767*32767  OutDataTypeStr=int32
  Data Store Read1 : DataStoreRead  DataStoreName=Ts_Point  IndexOptions=Index vector (dialog)  Indices=1  OutputSizes=1
  Data Store Read3 : DataStoreRead  DataStoreName=Curr_Limit  IndexOptions=Index vector (dialog)  Indices=1  OutputSizes=1
  Data Type Conversion3 : DataTypeConversion  Commented=on  OutDataTypeStr=int16  SaturateOnIntegerOverflow=off
  Divide : Product  Commented=on  Inputs=*/  OutDataTypeStr=int32  RndMeth=Zero
  Gain : Gain  Gain=-1  OutDataTypeStr=int32  RndMeth=Zero
  Product1 : Product  OutDataTypeStr=int32  RndMeth=Zero
  Product2 : Product  OutDataTypeStr=int32  RndMeth=Zero
  Saturation Dynamic2 : simulink/Discontinuities/Saturation Dynamic  OutMin=[]  OutMax=[]  OutDataTypeStr=Inherit: Same as second input  OutDataType=fixdt(1, 16)  OutScaling=2^-10  RndMeth=Zero  DoSatur=off
  Shift Arithmetic : ArithShift  BitShiftNumberSource=Input port  BitShiftNumber=8  BitShiftDirection=Right
      settings: InputPortMap=u0,p1
  Sum : Sum  Inputs=|++  OutDataTypeStr=int32  RndMeth=Zero
  Sum2 : Sum  Inputs=-+  OutDataTypeStr=int32  RndMeth=Zero
  Ts适当放大的缩小系数， 详见初始化模块 : ArithShift  Commented=on  BitShiftNumber=TS_POINT_GAIN  DiagnosticForOORShift=Error
  Unit Delay : UnitDelay  SampleTime=-1  HasFrameUpgradeWarning=on
  周期定点化适当放大2^n : Constant  Value=TS_POINT_GAIN
  积分器运行频率 : Constant  Commented=on  Value=FOC_FRQ
  这个是缩小周期增益的 : ArithShift  BitShiftNumber=15  DiagnosticForOORShift=Error
  output : Outport
  wires:
  积分器运行频率/1 -> Data Type Conversion3/1
  Data Type Conversion3/1 -> Divide/2
  Product2/1 -> 这个是缩小周期增益的/1
  Ki/1 -> Shift Arithmetic/1
  Shift Arithmetic/1 -> Product1/1
  Data Store Read1/1 -> Product2/1
  input/1 -> Product2/2
  周期定点化适当放大2^n/1 -> Shift Arithmetic/2
  Constant/1 -> Sum2/2
  Data Store Read3/1 -> Sum2/1, [limit]
  Sum2/1 -> [Limit1]
  [limit] -> Gain/1
  Product1/1 -> Sum/1
  这个是缩小周期增益的/1 -> Product1/2
  Unit Delay/1 -> Sum/2
  Gain/1 -> Saturation Dynamic2/3
  Sum/1 -> Saturation Dynamic2/2
  [limit] -> Saturation Dynamic2/1
  Saturation Dynamic2/1 -> Unit Delay/1, output/1

== system Senorless/FOC_PointModel/idq_Controller/PI Controller1/积分器 ==
  Ki : Inport
  input : Inport  Port=2
  Constant : Constant  Value=32767*32767  OutDataTypeStr=int32
  Data Store Read1 : DataStoreRead  DataStoreName=Ts_Point  IndexOptions=Index vector (dialog)  Indices=1  OutputSizes=1
  Data Store Read3 : DataStoreRead  DataStoreName=Curr_Limit  IndexOptions=Index vector (dialog)  Indices=1  OutputSizes=1
  Data Type Conversion3 : DataTypeConversion  Commented=on  OutDataTypeStr=int16  SaturateOnIntegerOverflow=off
  Divide : Product  Commented=on  Inputs=*/  OutDataTypeStr=int32  RndMeth=Zero
  Gain : Gain  Gain=-1  OutDataTypeStr=int32  RndMeth=Zero
  Product1 : Product  OutDataTypeStr=int32  RndMeth=Zero
  Product2 : Product  OutDataTypeStr=int32  RndMeth=Zero
  Saturation Dynamic2 : simulink/Discontinuities/Saturation Dynamic  OutMin=[]  OutMax=[]  OutDataTypeStr=Inherit: Same as second input  OutDataType=fixdt(1, 16)  OutScaling=2^-10  RndMeth=Zero  DoSatur=off
  Shift Arithmetic : ArithShift  BitShiftNumberSource=Input port  BitShiftNumber=8  BitShiftDirection=Right
      settings: InputPortMap=u0,p1
  Sum : Sum  Inputs=|++  OutDataTypeStr=int32  RndMeth=Zero
  Sum2 : Sum  Inputs=-+  OutDataTypeStr=int32  RndMeth=Zero
  Ts适当放大的缩小系数， 详见初始化模块 : ArithShift  Commented=on  BitShiftNumber=TS_POINT_GAIN  DiagnosticForOORShift=Error
  Unit Delay : UnitDelay  SampleTime=-1  HasFrameUpgradeWarning=on
  周期定点化适当放大2^n : Constant  Value=TS_POINT_GAIN
  积分器运行频率 : Constant  Commented=on  Value=FOC_FRQ
  这个是缩小周期增益的 : ArithShift  BitShiftNumber=15  DiagnosticForOORShift=Error
  output : Outport
  wires:
  Saturation Dynamic2/1 -> output/1, Unit Delay/1
  [limit] -> Saturation Dynamic2/1
  Sum/1 -> Saturation Dynamic2/2
  Gain/1 -> Saturation Dynamic2/3
  Unit Delay/1 -> Sum/2
  这个是缩小周期增益的/1 -> Product1/2
  Product1/1 -> Sum/1
  [limit] -> Gain/1
  Sum2/1 -> [Limit1]
  Data Store Read3/1 -> [limit], Sum2/1
  Constant/1 -> Sum2/2
  周期定点化适当放大2^n/1 -> Shift Arithmetic/2
  input/1 -> Product2/2
  Data Store Read1/1 -> Product2/1
  Shift Arithmetic/1 -> Product1/1
  Ki/1 -> Shift Arithmetic/1
  Product2/1 -> 这个是缩小周期增益的/1
  Data Type Conversion3/1 -> Divide/2
  积分器运行频率/1 -> Data Type Conversion3/1
